simulink model "QueuingSys"  (R2019a)
settings: Solver=VariableStepAuto  StartTime=0.0  StopTime=100  RelTol=1e-3  EnableMultiTasking=on
undefined symbols (not defined in the file or in its folder): m, n
(part 1 of 5)
settings Model: Creator=The MathWorks, Inc.  LastModifiedBy=Mojzar
settings DataIOCC: LimitDataPoints=on  SaveFormat=Array  ReturnWorkspaceOutputs=off
settings OptimizationCC: LifeSpan=inf
settings DebuggingCC: AllowSymbolicDim=off  SFUnexpectedBacktrackingDiag=warning  SFNoUnconditionalDefaultTransitionDiag=warning  SFExecutionAtInitializationDiag=none  ArithmeticOperatorsInVariantConditions=warning
settings ModelReferenceCC: PropagateSignalLabelsOutOfModel=off
settings SFSimCC: SimUseLocalCustomCode=off
settings RTWCC: RTWUseLocalCustomCode=off
settings CodeAppCC: StateflowObjectComments=on
settings GRTTargetCC: TargetLangStandard=C89/C90 (ANSI)  GeneratePreprocessorConditionals=Disable all
settings ConfigComp: CovMetricSettings=dw  CovHtmlReporting=on  CovSaveCumulativeToWorkspaceVar=on  CovSaveSingleToWorkspaceVar=on  CovExternalEMLEnable=off  CovSFcnEnable=off

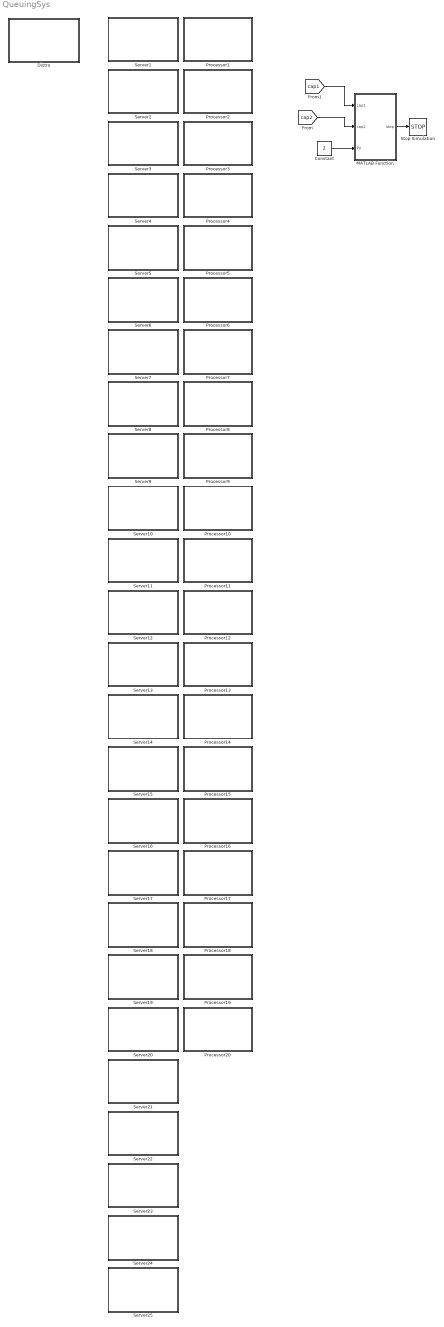
== system QueuingSys ==
  Constant : Constant  Value=2  SampleTime=-1
  Distro : Subsystem
  MATLAB Function : MATLAB Function  TreatAsAtomicUnit=on
  Processor1 : Subsystem
  Processor10 : Subsystem
  Processor11 : Subsystem
  Processor12 : Subsystem
  Processor13 : Subsystem
  Processor14 : Subsystem
  Processor15 : Subsystem
  Processor16 : Subsystem
  Processor17 : Subsystem
  Processor18 : Subsystem
  Processor19 : Subsystem
  Processor2 : Subsystem
  Processor20 : Subsystem
  Processor3 : Subsystem
  Processor4 : Subsystem
  Processor5 : Subsystem
  Processor6 : Subsystem
  Processor7 : Subsystem
  Processor8 : Subsystem
  Processor9 : Subsystem
  Server1 : Subsystem
  Server10 : Subsystem
  Server11 : Subsystem
  Server12 : Subsystem
  Server13 : Subsystem
  Server14 : Subsystem
  Server15 : Subsystem
  Server16 : Subsystem
  Server17 : Subsystem
  Server18 : Subsystem
  Server19 : Subsystem
  Server2 : Subsystem
  Server20 : Subsystem
  Server21 : Subsystem
  Server22 : Subsystem
  Server23 : Subsystem
  Server24 : Subsystem
  Server25 : Subsystem
  Server3 : Subsystem
  Server4 : Subsystem
  Server5 : Subsystem
  Server6 : Subsystem
  Server7 : Subsystem
  Server8 : Subsystem
  Server9 : Subsystem
  Stop Simulation : Stop
  wires:
  [cap2] -> MATLAB Function/2(cap2)
  [cap1] -> MATLAB Function/1(cap1)
  MATLAB Function/1(stop) -> Stop Simulation/1
  Constant/1 -> MATLAB Function/3(Pn)

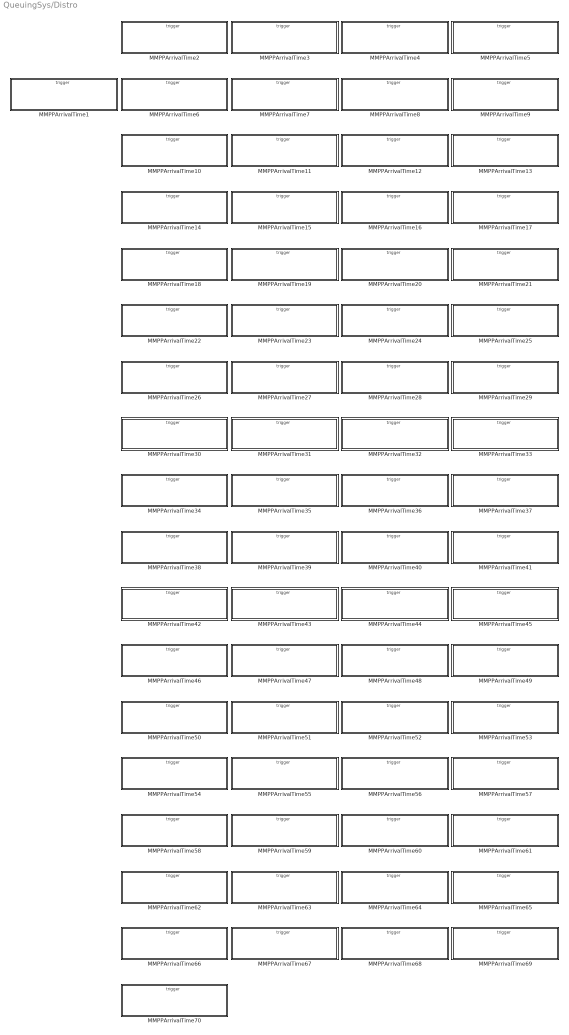
== system QueuingSys/Distro ==
  MMPPArrivalTime1 : Subsystem  TreatAsAtomicUnit=on
  MMPPArrivalTime10 : Subsystem  TreatAsAtomicUnit=on
  MMPPArrivalTime11 : Subsystem  TreatAsAtomicUnit=on
  MMPPArrivalTime12 : Subsystem  TreatAsAtomicUnit=on
  MMPPArrivalTime13 : Subsystem  TreatAsAtomicUnit=on
  MMPPArrivalTime14 : Subsystem  TreatAsAtomicUnit=on
  MMPPArrivalTime15 : Subsystem  TreatAsAtomicUnit=on
  MMPPArrivalTime16 : Subsystem  TreatAsAtomicUnit=on
  MMPPArrivalTime17 : Subsystem  TreatAsAtomicUnit=on
  MMPPArrivalTime18 : Subsystem  TreatAsAtomicUnit=on
  MMPPArrivalTime19 : Subsystem  TreatAsAtomicUnit=on
  MMPPArrivalTime2 : Subsystem  TreatAsAtomicUnit=on
  MMPPArrivalTime20 : Subsystem  TreatAsAtomicUnit=on
  MMPPArrivalTime21 : Subsystem  TreatAsAtomicUnit=on
  MMPPArrivalTime22 : Subsystem  TreatAsAtomicUnit=on
  MMPPArrivalTime23 : Subsystem  TreatAsAtomicUnit=on
  MMPPArrivalTime24 : Subsystem  TreatAsAtomicUnit=on
  MMPPArrivalTime25 : Subsystem  TreatAsAtomicUnit=on
  MMPPArrivalTime26 : Subsystem  TreatAsAtomicUnit=on
  MMPPArrivalTime27 : Subsystem  TreatAsAtomicUnit=on
  MMPPArrivalTime28 : Subsystem  TreatAsAtomicUnit=on
  MMPPArrivalTime29 : Subsystem  TreatAsAtomicUnit=on
  MMPPArrivalTime3 : Subsystem  TreatAsAtomicUnit=on
  MMPPArrivalTime30 : Subsystem  TreatAsAtomicUnit=on
  MMPPArrivalTime31 : Subsystem  TreatAsAtomicUnit=on
  MMPPArrivalTime32 : Subsystem  TreatAsAtomicUnit=on
  MMPPArrivalTime33 : Subsystem  TreatAsAtomicUnit=on
  MMPPArrivalTime34 : Subsystem  TreatAsAtomicUnit=on
  MMPPArrivalTime35 : Subsystem  TreatAsAtomicUnit=on
  MMPPArrivalTime36 : Subsystem  TreatAsAtomicUnit=on
  MMPPArrivalTime37 : Subsystem  TreatAsAtomicUnit=on
  MMPPArrivalTime38 : Subsystem  TreatAsAtomicUnit=on
  MMPPArrivalTime39 : Subsystem  TreatAsAtomicUnit=on
  MMPPArrivalTime4 : Subsystem  TreatAsAtomicUnit=on
  MMPPArrivalTime40 : Subsystem  TreatAsAtomicUnit=on
  MMPPArrivalTime41 : Subsystem  TreatAsAtomicUnit=on
  MMPPArrivalTime42 : Subsystem  TreatAsAtomicUnit=on
  MMPPArrivalTime43 : Subsystem  TreatAsAtomicUnit=on
  MMPPArrivalTime44 : Subsystem  TreatAsAtomicUnit=on
  MMPPArrivalTime45 : Subsystem  TreatAsAtomicUnit=on
  MMPPArrivalTime46 : Subsystem  TreatAsAtomicUnit=on
  MMPPArrivalTime47 : Subsystem  TreatAsAtomicUnit=on
  MMPPArrivalTime48 : Subsystem  TreatAsAtomicUnit=on
  MMPPArrivalTime49 : Subsystem  TreatAsAtomicUnit=on
  MMPPArrivalTime5 : Subsystem  TreatAsAtomicUnit=on
  MMPPArrivalTime50 : Subsystem  TreatAsAtomicUnit=on
  MMPPArrivalTime51 : Subsystem  TreatAsAtomicUnit=on
  MMPPArrivalTime52 : Subsystem  TreatAsAtomicUnit=on
  MMPPArrivalTime53 : Subsystem  TreatAsAtomicUnit=on
  MMPPArrivalTime54 : Subsystem  TreatAsAtomicUnit=on
  MMPPArrivalTime55 : Subsystem  TreatAsAtomicUnit=on
  MMPPArrivalTime56 : Subsystem  TreatAsAtomicUnit=on
  MMPPArrivalTime57 : Subsystem  TreatAsAtomicUnit=on
  MMPPArrivalTime58 : Subsystem  TreatAsAtomicUnit=on
  MMPPArrivalTime59 : Subsystem  TreatAsAtomicUnit=on
  MMPPArrivalTime6 : Subsystem  TreatAsAtomicUnit=on
  MMPPArrivalTime60 : Subsystem  TreatAsAtomicUnit=on
  MMPPArrivalTime61 : Subsystem  TreatAsAtomicUnit=on
  MMPPArrivalTime62 : Subsystem  TreatAsAtomicUnit=on
  MMPPArrivalTime63 : Subsystem  TreatAsAtomicUnit=on
  MMPPArrivalTime64 : Subsystem  TreatAsAtomicUnit=on
  MMPPArrivalTime65 : Subsystem  TreatAsAtomicUnit=on
  MMPPArrivalTime66 : Subsystem  TreatAsAtomicUnit=on
  MMPPArrivalTime67 : Subsystem  TreatAsAtomicUnit=on
  MMPPArrivalTime68 : Subsystem  TreatAsAtomicUnit=on
  MMPPArrivalTime69 : Subsystem  TreatAsAtomicUnit=on
  MMPPArrivalTime7 : Subsystem  TreatAsAtomicUnit=on
  MMPPArrivalTime70 : Subsystem  TreatAsAtomicUnit=on
  MMPPArrivalTime8 : Subsystem  TreatAsAtomicUnit=on
  MMPPArrivalTime9 : Subsystem  TreatAsAtomicUnit=on

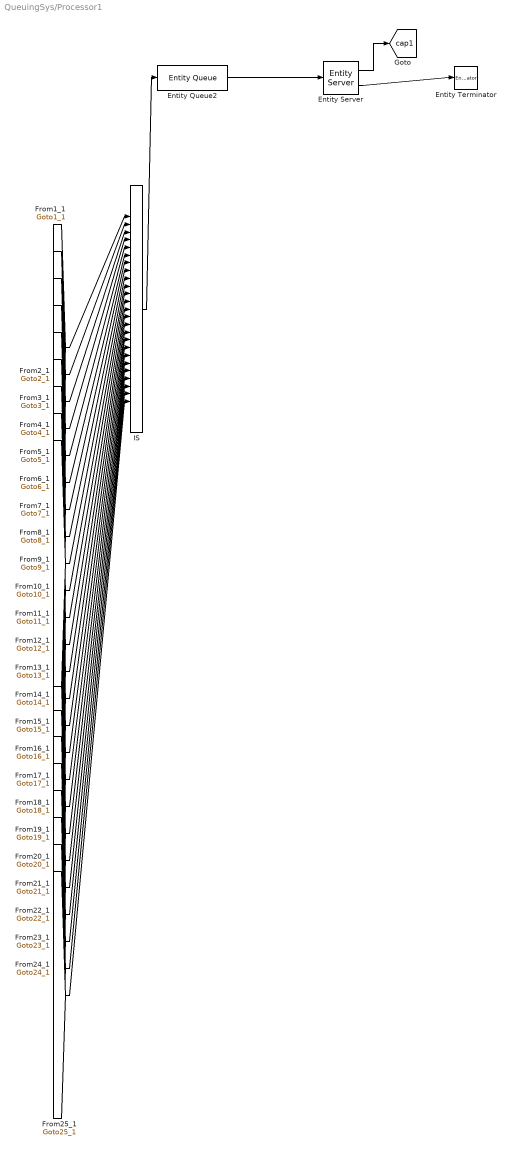
== system QueuingSys/Processor1 ==
  Entity Queue2 : EntityQueue  InputPortMessageModes=m  OutputPortMessageModes=m  Capacity=Inf  MulticastTag=B
      settings: OutputPortMap=o5
  Entity Server : EntityServer  InputPortMessageModes=m  OutputPortMessageModes=n,m  Capacity=4  ServiceTimeSource=MATLAB action  ServiceTimeAction=dt =MMPPArrivalTime51();  NumberEntitiesInBlock=on
      settings: OutputPortMap=o1,o9
  Entity Terminator : EntityTerminator  InputPortMessageModes=m
  IS : EntityInputSwitch  InputPortMessageModes=m,m,m,m,m,m,m,m,m,m,m,m,m,m,m,m,m,m,m,m,m,m,m,m,m  OutputPortMessageModes=m  NumberInputPorts=25
      settings: InputPortMap=u1,u2,u3,u4,u5,u6,u7,u8,u9,u10,u11,u12,u13,u14,u15,u16,u17,u18,u19,u20,u21,u22,u23,u24,u25
  tag scope: cap1=global
  wires:
  IS/1 -> Entity Queue2/1
  Entity Server/2 -> Entity Terminator/1
  Entity Queue2/1 -> Entity Server/1
  [Goto1_1] -> IS/1
  [Goto2_1] -> IS/2
  [Goto3_1] -> IS/3
  [Goto4_1] -> IS/4
  [Goto5_1] -> IS/5
  [Goto6_1] -> IS/6
  [Goto7_1] -> IS/7
  [Goto8_1] -> IS/8
  [Goto9_1] -> IS/9
  [Goto10_1] -> IS/10
  [Goto11_1] -> IS/11
  [Goto12_1] -> IS/12
  [Goto13_1] -> IS/13
  [Goto14_1] -> IS/14
  [Goto15_1] -> IS/15
  [Goto16_1] -> IS/16
  [Goto17_1] -> IS/17
  [Goto18_1] -> IS/18
  [Goto19_1] -> IS/19
  [Goto20_1] -> IS/20
  [Goto21_1] -> IS/21
  [Goto22_1] -> IS/22
  [Goto23_1] -> IS/23
  [Goto24_1] -> IS/24
  [Goto25_1] -> IS/25
  Entity Server/1 -> [cap1]

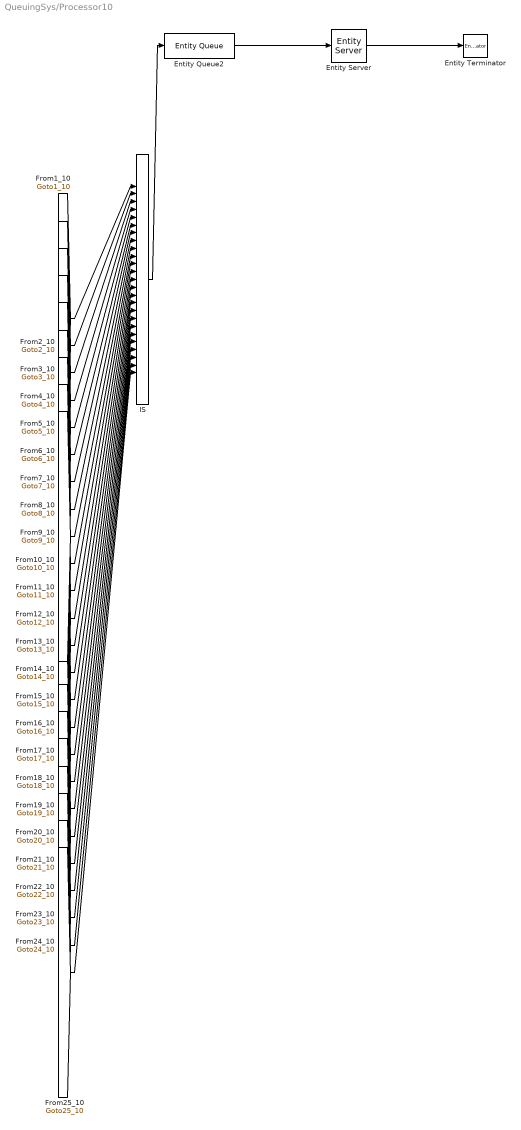
== system QueuingSys/Processor10 ==
  Entity Queue2 : EntityQueue  InputPortMessageModes=m  OutputPortMessageModes=m  Capacity=Inf  MulticastTag=B
      settings: OutputPortMap=o5
  Entity Server : EntityServer  InputPortMessageModes=m  OutputPortMessageModes=m  Capacity=3  ServiceTimeSource=MATLAB action  ServiceTimeAction=dt =MMPPArrivalTime60();
  Entity Terminator : EntityTerminator  InputPortMessageModes=m
  IS : EntityInputSwitch  InputPortMessageModes=m,m,m,m,m,m,m,m,m,m,m,m,m,m,m,m,m,m,m,m,m,m,m,m,m  OutputPortMessageModes=m  NumberInputPorts=25
      settings: InputPortMap=u1,u2,u3,u4,u5,u6,u7,u8,u9,u10,u11,u12,u13,u14,u15,u16,u17,u18,u19,u20,u21,u22,u23,u24,u25
  wires:
  Entity Queue2/1 -> Entity Server/1
  Entity Server/1 -> Entity Terminator/1
  IS/1 -> Entity Queue2/1
  [Goto1_10] -> IS/1
  [Goto2_10] -> IS/2
  [Goto3_10] -> IS/3
  [Goto4_10] -> IS/4
  [Goto5_10] -> IS/5
  [Goto6_10] -> IS/6
  [Goto7_10] -> IS/7
  [Goto8_10] -> IS/8
  [Goto9_10] -> IS/9
  [Goto10_10] -> IS/10
  [Goto11_10] -> IS/11
  [Goto12_10] -> IS/12
  [Goto13_10] -> IS/13
  [Goto14_10] -> IS/14
  [Goto15_10] -> IS/15
  [Goto16_10] -> IS/16
  [Goto17_10] -> IS/17
  [Goto18_10] -> IS/18
  [Goto19_10] -> IS/19
  [Goto20_10] -> IS/20
  [Goto21_10] -> IS/21
  [Goto22_10] -> IS/22
  [Goto23_10] -> IS/23
  [Goto24_10] -> IS/24
  [Goto25_10] -> IS/25

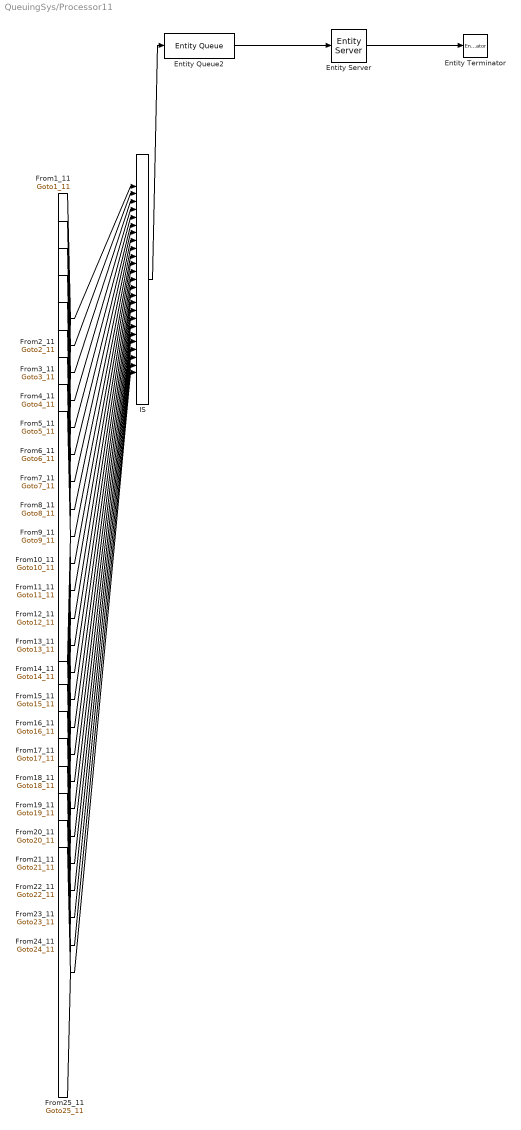
== system QueuingSys/Processor11 ==
  Entity Queue2 : EntityQueue  InputPortMessageModes=m  OutputPortMessageModes=m  Capacity=Inf  MulticastTag=B
      settings: OutputPortMap=o5
  Entity Server : EntityServer  InputPortMessageModes=m  OutputPortMessageModes=m  Capacity=3  ServiceTimeSource=MATLAB action  ServiceTimeAction=dt =MMPPArrivalTime61();
  Entity Terminator : EntityTerminator  InputPortMessageModes=m
  IS : EntityInputSwitch  InputPortMessageModes=m,m,m,m,m,m,m,m,m,m,m,m,m,m,m,m,m,m,m,m,m,m,m,m,m  OutputPortMessageModes=m  NumberInputPorts=25
      settings: InputPortMap=u1,u2,u3,u4,u5,u6,u7,u8,u9,u10,u11,u12,u13,u14,u15,u16,u17,u18,u19,u20,u21,u22,u23,u24,u25
  wires:
  IS/1 -> Entity Queue2/1
  Entity Server/1 -> Entity Terminator/1
  Entity Queue2/1 -> Entity Server/1
  [Goto1_11] -> IS/1
  [Goto2_11] -> IS/2
  [Goto3_11] -> IS/3
  [Goto4_11] -> IS/4
  [Goto5_11] -> IS/5
  [Goto6_11] -> IS/6
  [Goto7_11] -> IS/7
  [Goto8_11] -> IS/8
  [Goto9_11] -> IS/9
  [Goto10_11] -> IS/10
  [Goto11_11] -> IS/11
  [Goto12_11] -> IS/12
  [Goto13_11] -> IS/13
  [Goto14_11] -> IS/14
  [Goto15_11] -> IS/15
  [Goto16_11] -> IS/16
  [Goto17_11] -> IS/17
  [Goto18_11] -> IS/18
  [Goto19_11] -> IS/19
  [Goto20_11] -> IS/20
  [Goto21_11] -> IS/21
  [Goto22_11] -> IS/22
  [Goto23_11] -> IS/23
  [Goto24_11] -> IS/24
  [Goto25_11] -> IS/25

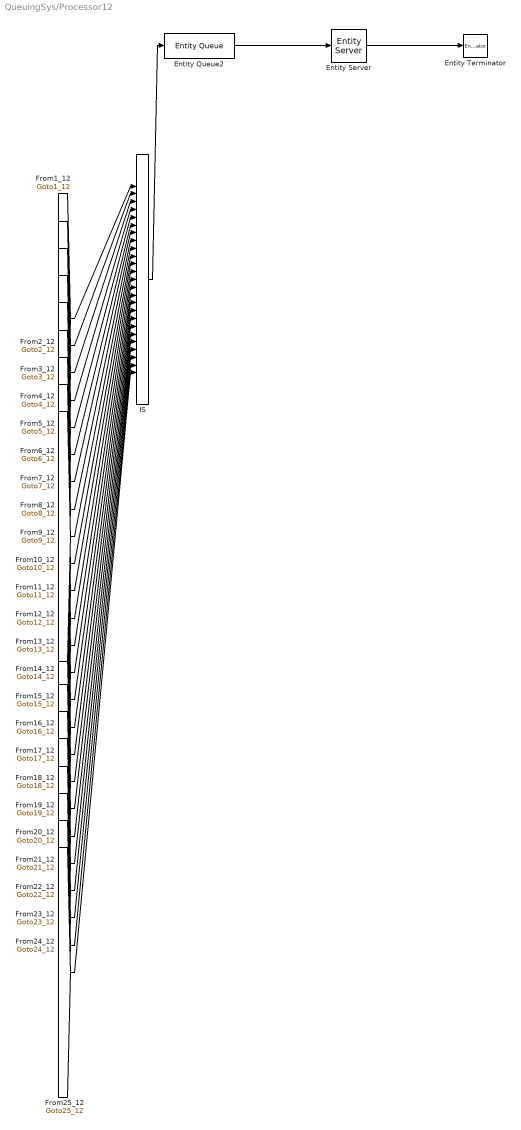
== system QueuingSys/Processor12 ==
  Entity Queue2 : EntityQueue  InputPortMessageModes=m  OutputPortMessageModes=m  Capacity=Inf  MulticastTag=B
      settings: OutputPortMap=o5
  Entity Server : EntityServer  InputPortMessageModes=m  OutputPortMessageModes=m  ServiceTimeSource=MATLAB action  ServiceTimeAction=dt =MMPPArrivalTime62();
  Entity Terminator : EntityTerminator  InputPortMessageModes=m
  IS : EntityInputSwitch  InputPortMessageModes=m,m,m,m,m,m,m,m,m,m,m,m,m,m,m,m,m,m,m,m,m,m,m,m,m  OutputPortMessageModes=m  NumberInputPorts=25
      settings: InputPortMap=u1,u2,u3,u4,u5,u6,u7,u8,u9,u10,u11,u12,u13,u14,u15,u16,u17,u18,u19,u20,u21,u22,u23,u24,u25
  wires:
  Entity Queue2/1 -> Entity Server/1
  Entity Server/1 -> Entity Terminator/1
  IS/1 -> Entity Queue2/1
  [Goto1_12] -> IS/1
  [Goto2_12] -> IS/2
  [Goto3_12] -> IS/3
  [Goto4_12] -> IS/4
  [Goto5_12] -> IS/5
  [Goto6_12] -> IS/6
  [Goto7_12] -> IS/7
  [Goto8_12] -> IS/8
  [Goto9_12] -> IS/9
  [Goto10_12] -> IS/10
  [Goto11_12] -> IS/11
  [Goto12_12] -> IS/12
  [Goto13_12] -> IS/13
  [Goto14_12] -> IS/14
  [Goto15_12] -> IS/15
  [Goto16_12] -> IS/16
  [Goto17_12] -> IS/17
  [Goto18_12] -> IS/18
  [Goto19_12] -> IS/19
  [Goto20_12] -> IS/20
  [Goto21_12] -> IS/21
  [Goto22_12] -> IS/22
  [Goto23_12] -> IS/23
  [Goto24_12] -> IS/24
  [Goto25_12] -> IS/25

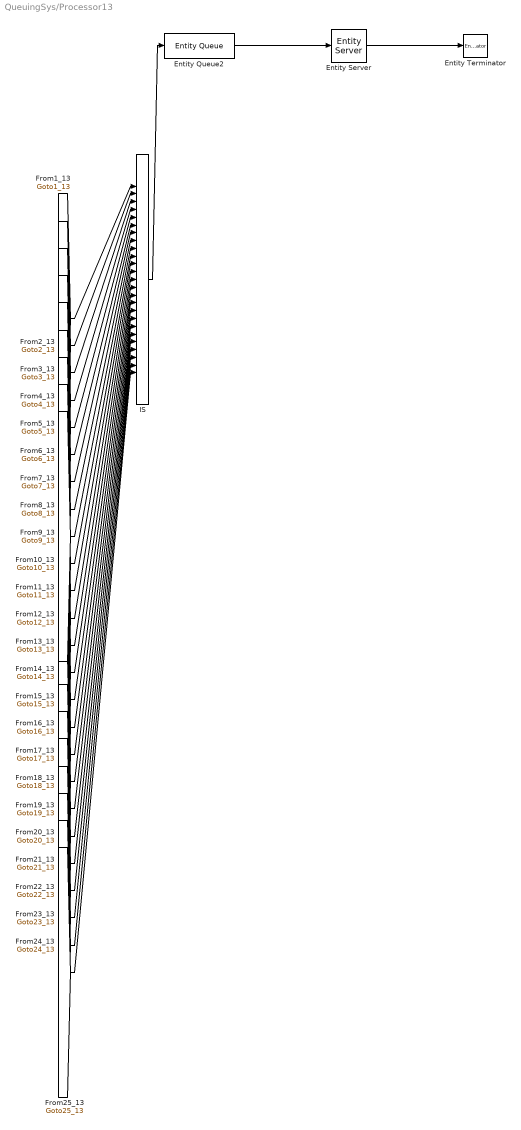
== system QueuingSys/Processor13 ==
  Entity Queue2 : EntityQueue  InputPortMessageModes=m  OutputPortMessageModes=m  Capacity=Inf  MulticastTag=B
      settings: OutputPortMap=o5
  Entity Server : EntityServer  InputPortMessageModes=m  OutputPortMessageModes=m  Capacity=4  ServiceTimeSource=MATLAB action  ServiceTimeAction=dt =MMPPArrivalTime63();
  Entity Terminator : EntityTerminator  InputPortMessageModes=m
  IS : EntityInputSwitch  InputPortMessageModes=m,m,m,m,m,m,m,m,m,m,m,m,m,m,m,m,m,m,m,m,m,m,m,m,m  OutputPortMessageModes=m  NumberInputPorts=25
      settings: InputPortMap=u1,u2,u3,u4,u5,u6,u7,u8,u9,u10,u11,u12,u13,u14,u15,u16,u17,u18,u19,u20,u21,u22,u23,u24,u25
  wires:
  IS/1 -> Entity Queue2/1
  Entity Server/1 -> Entity Terminator/1
  Entity Queue2/1 -> Entity Server/1
  [Goto1_13] -> IS/1
  [Goto2_13] -> IS/2
  [Goto3_13] -> IS/3
  [Goto4_13] -> IS/4
  [Goto5_13] -> IS/5
  [Goto6_13] -> IS/6
  [Goto7_13] -> IS/7
  [Goto8_13] -> IS/8
  [Goto9_13] -> IS/9
  [Goto10_13] -> IS/10
  [Goto11_13] -> IS/11
  [Goto12_13] -> IS/12
  [Goto13_13] -> IS/13
  [Goto14_13] -> IS/14
  [Goto15_13] -> IS/15
  [Goto16_13] -> IS/16
  [Goto17_13] -> IS/17
  [Goto18_13] -> IS/18
  [Goto19_13] -> IS/19
  [Goto20_13] -> IS/20
  [Goto21_13] -> IS/21
  [Goto22_13] -> IS/22
  [Goto23_13] -> IS/23
  [Goto24_13] -> IS/24
  [Goto25_13] -> IS/25

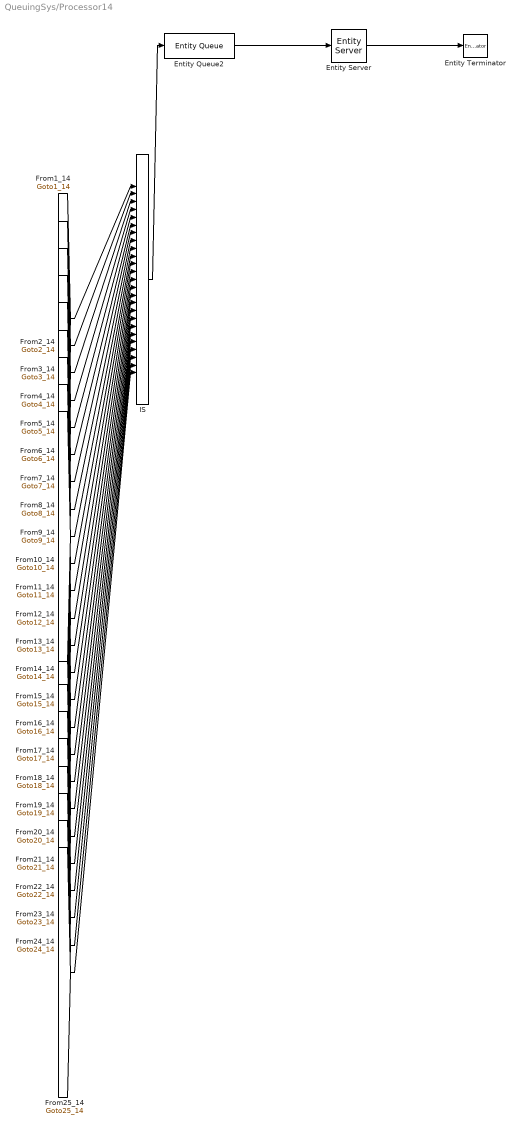
== system QueuingSys/Processor14 ==
  Entity Queue2 : EntityQueue  InputPortMessageModes=m  OutputPortMessageModes=m  Capacity=Inf  MulticastTag=B
      settings: OutputPortMap=o5
  Entity Server : EntityServer  InputPortMessageModes=m  OutputPortMessageModes=m  Capacity=4  ServiceTimeSource=MATLAB action  ServiceTimeAction=dt =MMPPArrivalTime64();
  Entity Terminator : EntityTerminator  InputPortMessageModes=m
  IS : EntityInputSwitch  InputPortMessageModes=m,m,m,m,m,m,m,m,m,m,m,m,m,m,m,m,m,m,m,m,m,m,m,m,m  OutputPortMessageModes=m  NumberInputPorts=25
      settings: InputPortMap=u1,u2,u3,u4,u5,u6,u7,u8,u9,u10,u11,u12,u13,u14,u15,u16,u17,u18,u19,u20,u21,u22,u23,u24,u25
  wires:
  Entity Queue2/1 -> Entity Server/1
  Entity Server/1 -> Entity Terminator/1
  IS/1 -> Entity Queue2/1
  [Goto1_14] -> IS/1
  [Goto2_14] -> IS/2
  [Goto3_14] -> IS/3
  [Goto4_14] -> IS/4
  [Goto5_14] -> IS/5
  [Goto6_14] -> IS/6
  [Goto7_14] -> IS/7
  [Goto8_14] -> IS/8
  [Goto9_14] -> IS/9
  [Goto10_14] -> IS/10
  [Goto11_14] -> IS/11
  [Goto12_14] -> IS/12
  [Goto13_14] -> IS/13
  [Goto14_14] -> IS/14
  [Goto15_14] -> IS/15
  [Goto16_14] -> IS/16
  [Goto17_14] -> IS/17
  [Goto18_14] -> IS/18
  [Goto19_14] -> IS/19
  [Goto20_14] -> IS/20
  [Goto21_14] -> IS/21
  [Goto22_14] -> IS/22
  [Goto23_14] -> IS/23
  [Goto24_14] -> IS/24
  [Goto25_14] -> IS/25

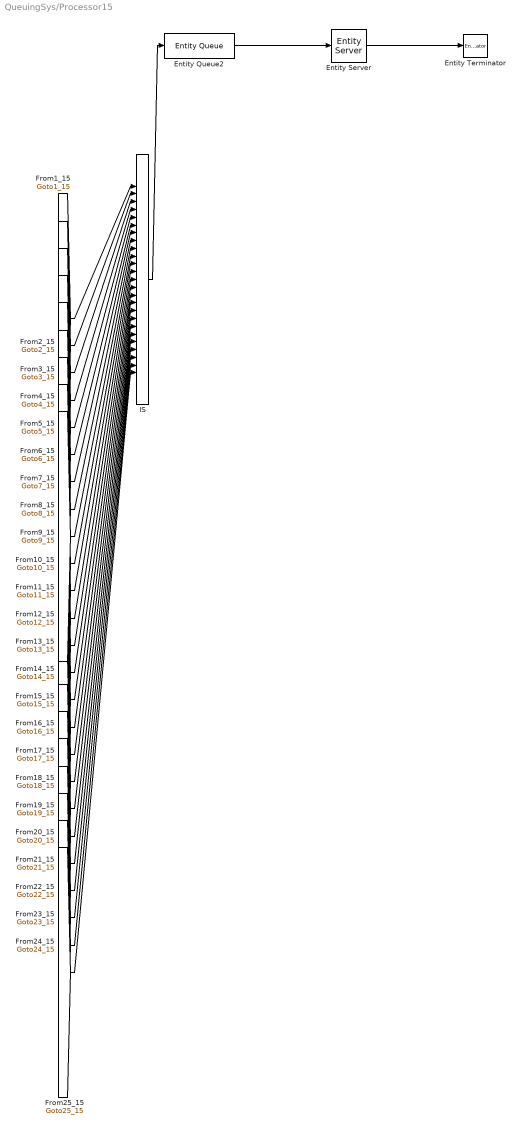
== system QueuingSys/Processor15 ==
  Entity Queue2 : EntityQueue  InputPortMessageModes=m  OutputPortMessageModes=m  Capacity=Inf  MulticastTag=B
      settings: OutputPortMap=o5
  Entity Server : EntityServer  InputPortMessageModes=m  OutputPortMessageModes=m  ServiceTimeSource=MATLAB action  ServiceTimeAction=dt =MMPPArrivalTime65();
  Entity Terminator : EntityTerminator  InputPortMessageModes=m
  IS : EntityInputSwitch  InputPortMessageModes=m,m,m,m,m,m,m,m,m,m,m,m,m,m,m,m,m,m,m,m,m,m,m,m,m  OutputPortMessageModes=m  NumberInputPorts=25
      settings: InputPortMap=u1,u2,u3,u4,u5,u6,u7,u8,u9,u10,u11,u12,u13,u14,u15,u16,u17,u18,u19,u20,u21,u22,u23,u24,u25
  wires:
  IS/1 -> Entity Queue2/1
  Entity Server/1 -> Entity Terminator/1
  Entity Queue2/1 -> Entity Server/1
  [Goto1_15] -> IS/1
  [Goto2_15] -> IS/2
  [Goto3_15] -> IS/3
  [Goto4_15] -> IS/4
  [Goto5_15] -> IS/5
  [Goto6_15] -> IS/6
  [Goto7_15] -> IS/7
  [Goto8_15] -> IS/8
  [Goto9_15] -> IS/9
  [Goto10_15] -> IS/10
  [Goto11_15] -> IS/11
  [Goto12_15] -> IS/12
  [Goto13_15] -> IS/13
  [Goto14_15] -> IS/14
  [Goto15_15] -> IS/15
  [Goto16_15] -> IS/16
  [Goto17_15] -> IS/17
  [Goto18_15] -> IS/18
  [Goto19_15] -> IS/19
  [Goto20_15] -> IS/20
  [Goto21_15] -> IS/21
  [Goto22_15] -> IS/22
  [Goto23_15] -> IS/23
  [Goto24_15] -> IS/24
  [Goto25_15] -> IS/25

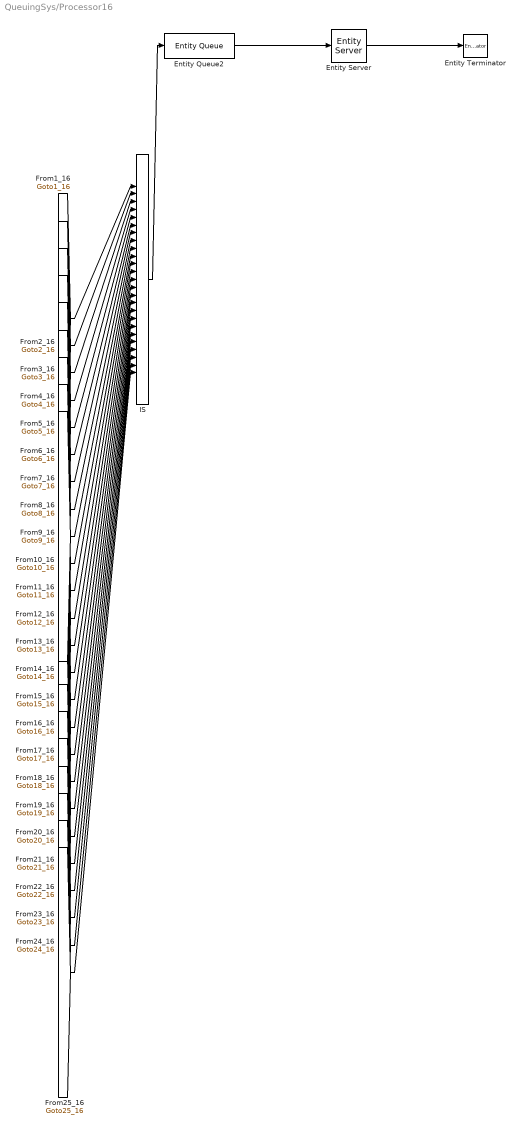
== system QueuingSys/Processor16 ==
  Entity Queue2 : EntityQueue  InputPortMessageModes=m  OutputPortMessageModes=m  Capacity=Inf  MulticastTag=B
      settings: OutputPortMap=o5
  Entity Server : EntityServer  InputPortMessageModes=m  OutputPortMessageModes=m  Capacity=1  ServiceTimeSource=MATLAB action  ServiceTimeAction=dt =MMPPArrivalTime66();
  Entity Terminator : EntityTerminator  InputPortMessageModes=m
  IS : EntityInputSwitch  InputPortMessageModes=m,m,m,m,m,m,m,m,m,m,m,m,m,m,m,m,m,m,m,m,m,m,m,m,m  OutputPortMessageModes=m  NumberInputPorts=25
      settings: InputPortMap=u1,u2,u3,u4,u5,u6,u7,u8,u9,u10,u11,u12,u13,u14,u15,u16,u17,u18,u19,u20,u21,u22,u23,u24,u25
  wires:
  Entity Queue2/1 -> Entity Server/1
  Entity Server/1 -> Entity Terminator/1
  IS/1 -> Entity Queue2/1
  [Goto1_16] -> IS/1
  [Goto2_16] -> IS/2
  [Goto3_16] -> IS/3
  [Goto4_16] -> IS/4
  [Goto5_16] -> IS/5
  [Goto6_16] -> IS/6
  [Goto7_16] -> IS/7
  [Goto8_16] -> IS/8
  [Goto9_16] -> IS/9
  [Goto10_16] -> IS/10
  [Goto11_16] -> IS/11
  [Goto12_16] -> IS/12
  [Goto13_16] -> IS/13
  [Goto14_16] -> IS/14
  [Goto15_16] -> IS/15
  [Goto16_16] -> IS/16
  [Goto17_16] -> IS/17
  [Goto18_16] -> IS/18
  [Goto19_16] -> IS/19
  [Goto20_16] -> IS/20
  [Goto21_16] -> IS/21
  [Goto22_16] -> IS/22
  [Goto23_16] -> IS/23
  [Goto24_16] -> IS/24
  [Goto25_16] -> IS/25

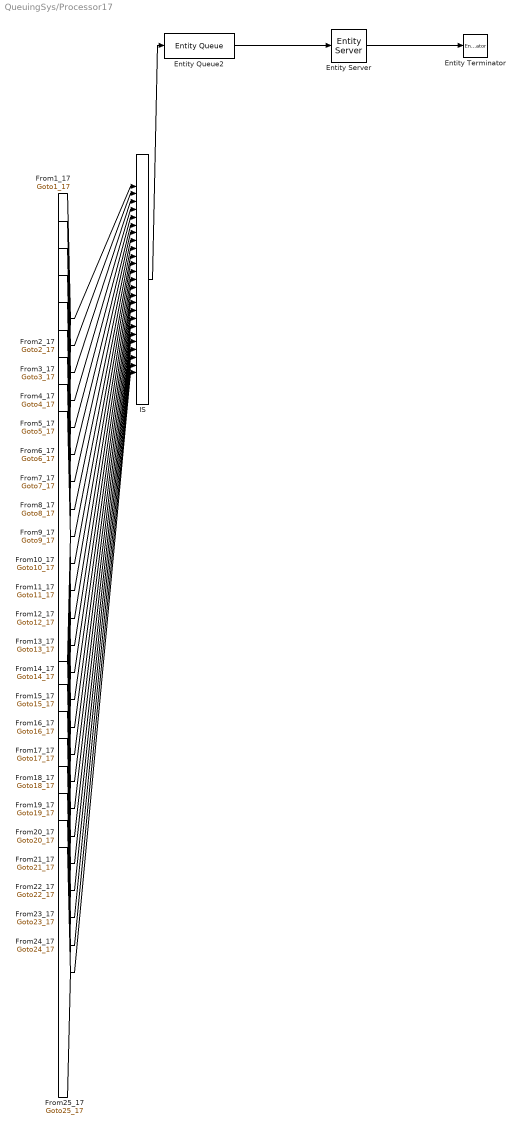
== system QueuingSys/Processor17 ==
  Entity Queue2 : EntityQueue  InputPortMessageModes=m  OutputPortMessageModes=m  Capacity=Inf  MulticastTag=B
      settings: OutputPortMap=o5
  Entity Server : EntityServer  InputPortMessageModes=m  OutputPortMessageModes=m  Capacity=2  ServiceTimeSource=MATLAB action  ServiceTimeAction=dt =MMPPArrivalTime67();
  Entity Terminator : EntityTerminator  InputPortMessageModes=m
  IS : EntityInputSwitch  InputPortMessageModes=m,m,m,m,m,m,m,m,m,m,m,m,m,m,m,m,m,m,m,m,m,m,m,m,m  OutputPortMessageModes=m  NumberInputPorts=25
      settings: InputPortMap=u1,u2,u3,u4,u5,u6,u7,u8,u9,u10,u11,u12,u13,u14,u15,u16,u17,u18,u19,u20,u21,u22,u23,u24,u25
  wires:
  IS/1 -> Entity Queue2/1
  Entity Server/1 -> Entity Terminator/1
  Entity Queue2/1 -> Entity Server/1
  [Goto1_17] -> IS/1
  [Goto2_17] -> IS/2
  [Goto3_17] -> IS/3
  [Goto4_17] -> IS/4
  [Goto5_17] -> IS/5
  [Goto6_17] -> IS/6
  [Goto7_17] -> IS/7
  [Goto8_17] -> IS/8
  [Goto9_17] -> IS/9
  [Goto10_17] -> IS/10
  [Goto11_17] -> IS/11
  [Goto12_17] -> IS/12
  [Goto13_17] -> IS/13
  [Goto14_17] -> IS/14
  [Goto15_17] -> IS/15
  [Goto16_17] -> IS/16
  [Goto17_17] -> IS/17
  [Goto18_17] -> IS/18
  [Goto19_17] -> IS/19
  [Goto20_17] -> IS/20
  [Goto21_17] -> IS/21
  [Goto22_17] -> IS/22
  [Goto23_17] -> IS/23
  [Goto24_17] -> IS/24
  [Goto25_17] -> IS/25

== system QueuingSys/Processor18 ==
  Entity Queue2 : EntityQueue  InputPortMessageModes=m  OutputPortMessageModes=m  Capacity=Inf  MulticastTag=B
      settings: OutputPortMap=o5
  Entity Server : EntityServer  InputPortMessageModes=m  OutputPortMessageModes=m  Capacity=7  ServiceTimeSource=MATLAB action  ServiceTimeAction=dt =MMPPArrivalTime68();
  Entity Terminator : EntityTerminator  InputPortMessageModes=m
  IS : EntityInputSwitch  InputPortMessageModes=m,m,m,m,m,m,m,m,m,m,m,m,m,m,m,m,m,m,m,m,m,m,m,m,m  OutputPortMessageModes=m  NumberInputPorts=25
      settings: InputPortMap=u1,u2,u3,u4,u5,u6,u7,u8,u9,u10,u11,u12,u13,u14,u15,u16,u17,u18,u19,u20,u21,u22,u23,u24,u25
  wires:
  Entity Queue2/1 -> Entity Server/1
  Entity Server/1 -> Entity Terminator/1
  IS/1 -> Entity Queue2/1
  [Goto1_18] -> IS/1
  [Goto2_18] -> IS/2
  [Goto3_18] -> IS/3
  [Goto4_18] -> IS/4
  [Goto5_18] -> IS/5
  [Goto6_18] -> IS/6
  [Goto7_18] -> IS/7
  [Goto8_18] -> IS/8
  [Goto9_18] -> IS/9
  [Goto10_18] -> IS/10
  [Goto11_18] -> IS/11
  [Goto12_18] -> IS/12
  [Goto13_18] -> IS/13
  [Goto14_18] -> IS/14
  [Goto15_18] -> IS/15
  [Goto16_18] -> IS/16
  [Goto17_18] -> IS/17
  [Goto18_18] -> IS/18
  [Goto19_18] -> IS/19
  [Goto20_18] -> IS/20
  [Goto21_18] -> IS/21
  [Goto22_18] -> IS/22
  [Goto23_18] -> IS/23
  [Goto24_18] -> IS/24
  [Goto25_18] -> IS/25

== system QueuingSys/Processor19 ==
  Entity Queue2 : EntityQueue  InputPortMessageModes=m  OutputPortMessageModes=m  Capacity=Inf  MulticastTag=B
      settings: OutputPortMap=o5
  Entity Server : EntityServer  InputPortMessageModes=m  OutputPortMessageModes=m  ServiceTimeSource=MATLAB action  ServiceTimeAction=dt =MMPPArrivalTime69();
  Entity Terminator : EntityTerminator  InputPortMessageModes=m
  IS : EntityInputSwitch  InputPortMessageModes=m,m,m,m,m,m,m,m,m,m,m,m,m,m,m,m,m,m,m,m,m,m,m,m,m  OutputPortMessageModes=m  NumberInputPorts=25
      settings: InputPortMap=u1,u2,u3,u4,u5,u6,u7,u8,u9,u10,u11,u12,u13,u14,u15,u16,u17,u18,u19,u20,u21,u22,u23,u24,u25
  wires:
  IS/1 -> Entity Queue2/1
  Entity Server/1 -> Entity Terminator/1
  Entity Queue2/1 -> Entity Server/1
  [Goto1_19] -> IS/1
  [Goto2_19] -> IS/2
  [Goto3_19] -> IS/3
  [Goto4_19] -> IS/4
  [Goto5_19] -> IS/5
  [Goto6_19] -> IS/6
  [Goto7_19] -> IS/7
  [Goto8_19] -> IS/8
  [Goto9_19] -> IS/9
  [Goto10_19] -> IS/10
  [Goto11_19] -> IS/11
  [Goto12_19] -> IS/12
  [Goto13_19] -> IS/13
  [Goto14_19] -> IS/14
  [Goto15_19] -> IS/15
  [Goto16_19] -> IS/16
  [Goto17_19] -> IS/17
  [Goto18_19] -> IS/18
  [Goto19_19] -> IS/19
  [Goto20_19] -> IS/20
  [Goto21_19] -> IS/21
  [Goto22_19] -> IS/22
  [Goto23_19] -> IS/23
  [Goto24_19] -> IS/24
  [Goto25_19] -> IS/25

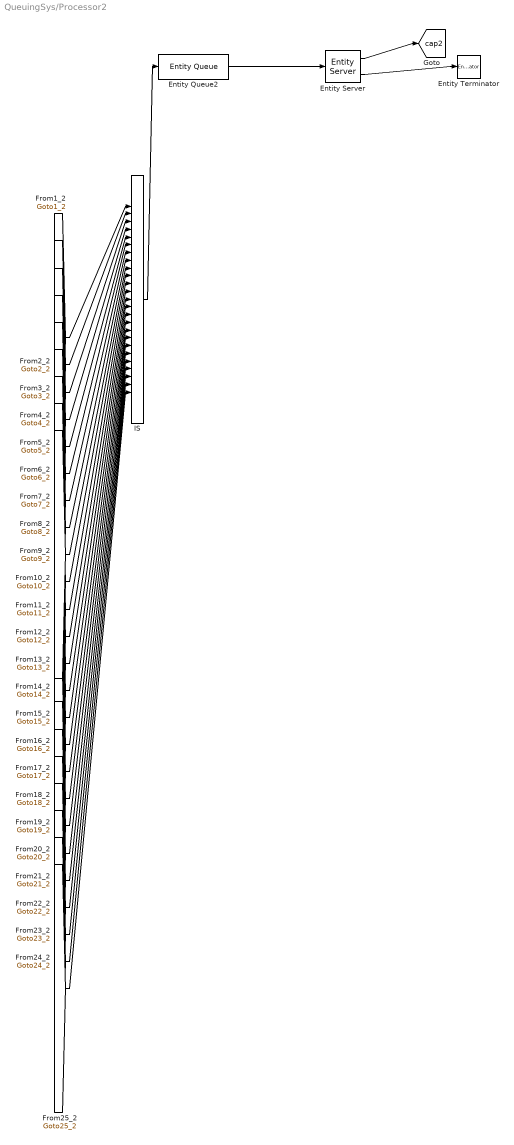
== system QueuingSys/Processor2 ==
  Entity Queue2 : EntityQueue  InputPortMessageModes=m  OutputPortMessageModes=m  Capacity=Inf  MulticastTag=B
      settings: OutputPortMap=o5
  Entity Server : EntityServer  InputPortMessageModes=m  OutputPortMessageModes=n,m  Capacity=3  ServiceTimeSource=MATLAB action  ServiceTimeAction=dt =MMPPArrivalTime52();  NumberEntitiesInBlock=on
      settings: OutputPortMap=o1,o9
  Entity Terminator : EntityTerminator  InputPortMessageModes=m
  IS : EntityInputSwitch  InputPortMessageModes=m,m,m,m,m,m,m,m,m,m,m,m,m,m,m,m,m,m,m,m,m,m,m,m,m  OutputPortMessageModes=m  NumberInputPorts=25
      settings: InputPortMap=u1,u2,u3,u4,u5,u6,u7,u8,u9,u10,u11,u12,u13,u14,u15,u16,u17,u18,u19,u20,u21,u22,u23,u24,u25
  tag scope: cap2=global
  wires:
  Entity Queue2/1 -> Entity Server/1
  Entity Server/2 -> Entity Terminator/1
  IS/1 -> Entity Queue2/1
  [Goto1_2] -> IS/1
  [Goto2_2] -> IS/2
  [Goto3_2] -> IS/3
  [Goto4_2] -> IS/4
  [Goto5_2] -> IS/5
  [Goto6_2] -> IS/6
  [Goto7_2] -> IS/7
  [Goto8_2] -> IS/8
  [Goto9_2] -> IS/9
  [Goto10_2] -> IS/10
  [Goto11_2] -> IS/11
  [Goto12_2] -> IS/12
  [Goto13_2] -> IS/13
  [Goto14_2] -> IS/14
  [Goto15_2] -> IS/15
  [Goto16_2] -> IS/16
  [Goto17_2] -> IS/17
  [Goto18_2] -> IS/18
  [Goto19_2] -> IS/19
  [Goto20_2] -> IS/20
  [Goto21_2] -> IS/21
  [Goto22_2] -> IS/22
  [Goto23_2] -> IS/23
  [Goto24_2] -> IS/24
  [Goto25_2] -> IS/25
  Entity Server/1 -> [cap2]

== system QueuingSys/Processor20 ==
  Entity Queue2 : EntityQueue  InputPortMessageModes=m  OutputPortMessageModes=m  Capacity=Inf  MulticastTag=B
      settings: OutputPortMap=o5
  Entity Server : EntityServer  InputPortMessageModes=m  OutputPortMessageModes=m  Capacity=1  ServiceTimeSource=MATLAB action  ServiceTimeAction=dt =MMPPArrivalTime70();
  Entity Terminator : EntityTerminator  InputPortMessageModes=m
  IS : EntityInputSwitch  InputPortMessageModes=m,m,m,m,m,m,m,m,m,m,m,m,m,m,m,m,m,m,m,m,m,m,m,m,m  OutputPortMessageModes=m  NumberInputPorts=25
      settings: InputPortMap=u1,u2,u3,u4,u5,u6,u7,u8,u9,u10,u11,u12,u13,u14,u15,u16,u17,u18,u19,u20,u21,u22,u23,u24,u25
  wires:
  Entity Queue2/1 -> Entity Server/1
  Entity Server/1 -> Entity Terminator/1
  IS/1 -> Entity Queue2/1
  [Goto1_20] -> IS/1
  [Goto2_20] -> IS/2
  [Goto3_20] -> IS/3
  [Goto4_20] -> IS/4
  [Goto5_20] -> IS/5
  [Goto6_20] -> IS/6
  [Goto7_20] -> IS/7
  [Goto8_20] -> IS/8
  [Goto9_20] -> IS/9
  [Goto10_20] -> IS/10
  [Goto11_20] -> IS/11
  [Goto12_20] -> IS/12
  [Goto13_20] -> IS/13
  [Goto14_20] -> IS/14
  [Goto15_20] -> IS/15
  [Goto16_20] -> IS/16
  [Goto17_20] -> IS/17
  [Goto18_20] -> IS/18
  [Goto19_20] -> IS/19
  [Goto20_20] -> IS/20
  [Goto21_20] -> IS/21
  [Goto22_20] -> IS/22
  [Goto23_20] -> IS/23
  [Goto24_20] -> IS/24
  [Goto25_20] -> IS/25

== system QueuingSys/Processor3 ==
  Entity Queue2 : EntityQueue  InputPortMessageModes=m  OutputPortMessageModes=m  Capacity=Inf  MulticastTag=B
      settings: OutputPortMap=o5
  Entity Server : EntityServer  InputPortMessageModes=m  OutputPortMessageModes=m  Capacity=2  ServiceTimeSource=MATLAB action  ServiceTimeAction=dt =MMPPArrivalTime53();
  Entity Terminator : EntityTerminator  InputPortMessageModes=m
  IS : EntityInputSwitch  InputPortMessageModes=m,m,m,m,m,m,m,m,m,m,m,m,m,m,m,m,m,m,m,m,m,m,m,m,m  OutputPortMessageModes=m  NumberInputPorts=25
      settings: InputPortMap=u1,u2,u3,u4,u5,u6,u7,u8,u9,u10,u11,u12,u13,u14,u15,u16,u17,u18,u19,u20,u21,u22,u23,u24,u25
  wires:
  IS/1 -> Entity Queue2/1
  Entity Server/1 -> Entity Terminator/1
  Entity Queue2/1 -> Entity Server/1
  [Goto1_3] -> IS/1
  [Goto2_3] -> IS/2
  [Goto3_3] -> IS/3
  [Goto4_3] -> IS/4
  [Goto5_3] -> IS/5
  [Goto6_3] -> IS/6
  [Goto7_3] -> IS/7
  [Goto8_3] -> IS/8
  [Goto9_3] -> IS/9
  [Goto10_3] -> IS/10
  [Goto11_3] -> IS/11
  [Goto12_3] -> IS/12
  [Goto13_3] -> IS/13
  [Goto14_3] -> IS/14
  [Goto15_3] -> IS/15
  [Goto16_3] -> IS/16
  [Goto17_3] -> IS/17
  [Goto18_3] -> IS/18
  [Goto19_3] -> IS/19
  [Goto20_3] -> IS/20
  [Goto21_3] -> IS/21
  [Goto22_3] -> IS/22
  [Goto23_3] -> IS/23
  [Goto24_3] -> IS/24
  [Goto25_3] -> IS/25

== system QueuingSys/Processor4 ==
  Entity Queue2 : EntityQueue  InputPortMessageModes=m  OutputPortMessageModes=m  Capacity=Inf  MulticastTag=B
      settings: OutputPortMap=o5
  Entity Server : EntityServer  InputPortMessageModes=m  OutputPortMessageModes=m  Capacity=3  ServiceTimeSource=MATLAB action  ServiceTimeAction=dt =MMPPArrivalTime54();
  Entity Terminator : EntityTerminator  InputPortMessageModes=m
  IS : EntityInputSwitch  InputPortMessageModes=m,m,m,m,m,m,m,m,m,m,m,m,m,m,m,m,m,m,m,m,m,m,m,m,m  OutputPortMessageModes=m  NumberInputPorts=25
      settings: InputPortMap=u1,u2,u3,u4,u5,u6,u7,u8,u9,u10,u11,u12,u13,u14,u15,u16,u17,u18,u19,u20,u21,u22,u23,u24,u25
  wires:
  Entity Queue2/1 -> Entity Server/1
  Entity Server/1 -> Entity Terminator/1
  IS/1 -> Entity Queue2/1
  [Goto1_4] -> IS/1
  [Goto2_4] -> IS/2
  [Goto3_4] -> IS/3
  [Goto4_4] -> IS/4
  [Goto5_4] -> IS/5
  [Goto6_4] -> IS/6
  [Goto7_4] -> IS/7
  [Goto8_4] -> IS/8
  [Goto9_4] -> IS/9
  [Goto10_4] -> IS/10
  [Goto11_4] -> IS/11
  [Goto12_4] -> IS/12
  [Goto13_4] -> IS/13
  [Goto14_4] -> IS/14
  [Goto15_4] -> IS/15
  [Goto16_4] -> IS/16
  [Goto17_4] -> IS/17
  [Goto18_4] -> IS/18
  [Goto19_4] -> IS/19
  [Goto20_4] -> IS/20
  [Goto21_4] -> IS/21
  [Goto22_4] -> IS/22
  [Goto23_4] -> IS/23
  [Goto24_4] -> IS/24
  [Goto25_4] -> IS/25

== system QueuingSys/Processor5 ==
  Entity Queue2 : EntityQueue  InputPortMessageModes=m  OutputPortMessageModes=m  Capacity=Inf  MulticastTag=B
      settings: OutputPortMap=o5
  Entity Server : EntityServer  InputPortMessageModes=m  OutputPortMessageModes=m  Capacity=6  ServiceTimeSource=MATLAB action  ServiceTimeAction=dt =MMPPArrivalTime55();
  Entity Terminator : EntityTerminator  InputPortMessageModes=m
  IS : EntityInputSwitch  InputPortMessageModes=m,m,m,m,m,m,m,m,m,m,m,m,m,m,m,m,m,m,m,m,m,m,m,m,m  OutputPortMessageModes=m  NumberInputPorts=25
      settings: InputPortMap=u1,u2,u3,u4,u5,u6,u7,u8,u9,u10,u11,u12,u13,u14,u15,u16,u17,u18,u19,u20,u21,u22,u23,u24,u25
  wires:
  IS/1 -> Entity Queue2/1
  Entity Server/1 -> Entity Terminator/1
  Entity Queue2/1 -> Entity Server/1
  [Goto1_5] -> IS/1
  [Goto2_5] -> IS/2
  [Goto3_5] -> IS/3
  [Goto4_5] -> IS/4
  [Goto5_5] -> IS/5
  [Goto6_5] -> IS/6
  [Goto7_5] -> IS/7
  [Goto8_5] -> IS/8
  [Goto9_5] -> IS/9
  [Goto10_5] -> IS/10
  [Goto11_5] -> IS/11
  [Goto12_5] -> IS/12
  [Goto13_5] -> IS/13
  [Goto14_5] -> IS/14
  [Goto15_5] -> IS/15
  [Goto16_5] -> IS/16
  [Goto17_5] -> IS/17
  [Goto18_5] -> IS/18
  [Goto19_5] -> IS/19
  [Goto20_5] -> IS/20
  [Goto21_5] -> IS/21
  [Goto22_5] -> IS/22
  [Goto23_5] -> IS/23
  [Goto24_5] -> IS/24
  [Goto25_5] -> IS/25

== system QueuingSys/Processor6 ==
  Entity Queue2 : EntityQueue  InputPortMessageModes=m  OutputPortMessageModes=m  Capacity=Inf  MulticastTag=B
      settings: OutputPortMap=o5
  Entity Server : EntityServer  InputPortMessageModes=m  OutputPortMessageModes=m  Capacity=6  ServiceTimeSource=MATLAB action  ServiceTimeAction=dt =MMPPArrivalTime56();
  Entity Terminator : EntityTerminator  InputPortMessageModes=m
  IS : EntityInputSwitch  InputPortMessageModes=m,m,m,m,m,m,m,m,m,m,m,m,m,m,m,m,m,m,m,m,m,m,m,m,m  OutputPortMessageModes=m  NumberInputPorts=25
      settings: InputPortMap=u1,u2,u3,u4,u5,u6,u7,u8,u9,u10,u11,u12,u13,u14,u15,u16,u17,u18,u19,u20,u21,u22,u23,u24,u25
  wires:
  Entity Queue2/1 -> Entity Server/1
  Entity Server/1 -> Entity Terminator/1
  IS/1 -> Entity Queue2/1
  [Goto1_6] -> IS/1
  [Goto2_6] -> IS/2
  [Goto3_6] -> IS/3
  [Goto4_6] -> IS/4
  [Goto5_6] -> IS/5
  [Goto6_6] -> IS/6
  [Goto7_6] -> IS/7
  [Goto8_6] -> IS/8
  [Goto9_6] -> IS/9
  [Goto10_6] -> IS/10
  [Goto11_6] -> IS/11
  [Goto12_6] -> IS/12
  [Goto13_6] -> IS/13
  [Goto14_6] -> IS/14
  [Goto15_6] -> IS/15
  [Goto16_6] -> IS/16
  [Goto17_6] -> IS/17
  [Goto18_6] -> IS/18
  [Goto19_6] -> IS/19
  [Goto20_6] -> IS/20
  [Goto21_6] -> IS/21
  [Goto22_6] -> IS/22
  [Goto23_6] -> IS/23
  [Goto24_6] -> IS/24
  [Goto25_6] -> IS/25

== system QueuingSys/Processor7 ==
  Entity Queue2 : EntityQueue  InputPortMessageModes=m  OutputPortMessageModes=m  Capacity=Inf  MulticastTag=B
      settings: OutputPortMap=o5
  Entity Server : EntityServer  InputPortMessageModes=m  OutputPortMessageModes=m  Capacity=7  ServiceTimeSource=MATLAB action  ServiceTimeAction=dt =MMPPArrivalTime57();
  Entity Terminator : EntityTerminator  InputPortMessageModes=m
  IS : EntityInputSwitch  InputPortMessageModes=m,m,m,m,m,m,m,m,m,m,m,m,m,m,m,m,m,m,m,m,m,m,m,m,m  OutputPortMessageModes=m  NumberInputPorts=25
      settings: InputPortMap=u1,u2,u3,u4,u5,u6,u7,u8,u9,u10,u11,u12,u13,u14,u15,u16,u17,u18,u19,u20,u21,u22,u23,u24,u25
  wires:
  IS/1 -> Entity Queue2/1
  Entity Server/1 -> Entity Terminator/1
  Entity Queue2/1 -> Entity Server/1
  [Goto1_7] -> IS/1
  [Goto2_7] -> IS/2
  [Goto3_7] -> IS/3
  [Goto4_7] -> IS/4
  [Goto5_7] -> IS/5
  [Goto6_7] -> IS/6
  [Goto7_7] -> IS/7
  [Goto8_7] -> IS/8
  [Goto9_7] -> IS/9
  [Goto10_7] -> IS/10
  [Goto11_7] -> IS/11
  [Goto12_7] -> IS/12
  [Goto13_7] -> IS/13
  [Goto14_7] -> IS/14
  [Goto15_7] -> IS/15
  [Goto16_7] -> IS/16
  [Goto17_7] -> IS/17
  [Goto18_7] -> IS/18
  [Goto19_7] -> IS/19
  [Goto20_7] -> IS/20
  [Goto21_7] -> IS/21
  [Goto22_7] -> IS/22
  [Goto23_7] -> IS/23
  [Goto24_7] -> IS/24
  [Goto25_7] -> IS/25

== system QueuingSys/Processor8 ==
  Entity Queue2 : EntityQueue  InputPortMessageModes=m  OutputPortMessageModes=m  Capacity=Inf  MulticastTag=B
      settings: OutputPortMap=o5
  Entity Server : EntityServer  InputPortMessageModes=m  OutputPortMessageModes=m  Capacity=4  ServiceTimeSource=MATLAB action  ServiceTimeAction=dt =MMPPArrivalTime58();
  Entity Terminator : EntityTerminator  InputPortMessageModes=m
  IS : EntityInputSwitch  InputPortMessageModes=m,m,m,m,m,m,m,m,m,m,m,m,m,m,m,m,m,m,m,m,m,m,m,m,m  OutputPortMessageModes=m  NumberInputPorts=25
      settings: InputPortMap=u1,u2,u3,u4,u5,u6,u7,u8,u9,u10,u11,u12,u13,u14,u15,u16,u17,u18,u19,u20,u21,u22,u23,u24,u25
  wires:
  Entity Queue2/1 -> Entity Server/1
  Entity Server/1 -> Entity Terminator/1
  IS/1 -> Entity Queue2/1
  [Goto1_8] -> IS/1
  [Goto2_8] -> IS/2
  [Goto3_8] -> IS/3
  [Goto4_8] -> IS/4
  [Goto5_8] -> IS/5
  [Goto6_8] -> IS/6
  [Goto7_8] -> IS/7
  [Goto8_8] -> IS/8
  [Goto9_8] -> IS/9
  [Goto10_8] -> IS/10
  [Goto11_8] -> IS/11
  [Goto12_8] -> IS/12
  [Goto13_8] -> IS/13
  [Goto14_8] -> IS/14
  [Goto15_8] -> IS/15
  [Goto16_8] -> IS/16
  [Goto17_8] -> IS/17
  [Goto18_8] -> IS/18
  [Goto19_8] -> IS/19
  [Goto20_8] -> IS/20
  [Goto21_8] -> IS/21
  [Goto22_8] -> IS/22
  [Goto23_8] -> IS/23
  [Goto24_8] -> IS/24
  [Goto25_8] -> IS/25

== system QueuingSys/Processor9 ==
  Entity Queue2 : EntityQueue  InputPortMessageModes=m  OutputPortMessageModes=m  Capacity=Inf  MulticastTag=B
      settings: OutputPortMap=o5
  Entity Server : EntityServer  InputPortMessageModes=m  OutputPortMessageModes=m  ServiceTimeSource=MATLAB action  ServiceTimeAction=dt =MMPPArrivalTime59();
  Entity Terminator : EntityTerminator  InputPortMessageModes=m
  IS : EntityInputSwitch  InputPortMessageModes=m,m,m,m,m,m,m,m,m,m,m,m,m,m,m,m,m,m,m,m,m,m,m,m,m  OutputPortMessageModes=m  NumberInputPorts=25
      settings: InputPortMap=u1,u2,u3,u4,u5,u6,u7,u8,u9,u10,u11,u12,u13,u14,u15,u16,u17,u18,u19,u20,u21,u22,u23,u24,u25
  wires:
  IS/1 -> Entity Queue2/1
  Entity Server/1 -> Entity Terminator/1
  Entity Queue2/1 -> Entity Server/1
  [Goto1_9] -> IS/1
  [Goto2_9] -> IS/2
  [Goto3_9] -> IS/3
  [Goto4_9] -> IS/4
  [Goto5_9] -> IS/5
  [Goto6_9] -> IS/6
  [Goto7_9] -> IS/7
  [Goto8_9] -> IS/8
  [Goto9_9] -> IS/9
  [Goto10_9] -> IS/10
  [Goto11_9] -> IS/11
  [Goto12_9] -> IS/12
  [Goto13_9] -> IS/13
  [Goto14_9] -> IS/14
  [Goto15_9] -> IS/15
  [Goto16_9] -> IS/16
  [Goto17_9] -> IS/17
  [Goto18_9] -> IS/18
  [Goto19_9] -> IS/19
  [Goto20_9] -> IS/20
  [Goto21_9] -> IS/21
  [Goto22_9] -> IS/22
  [Goto23_9] -> IS/23
  [Goto24_9] -> IS/24
  [Goto25_9] -> IS/25

== system QueuingSys/Server1 ==
  Entity Generator1 : EntityGenerator  OutputPortMessageModes=m  TimeSource=MATLAB action  IntergenerationTimeAction=dt =MMPPArrivalTime1();  EntityType=Structured  EntityTypeName=Entity
  Entity Queue1 : EntityQueue  InputPortMessageModes=m  OutputPortMessageModes=m  Capacity=Inf  MulticastTag=B
      settings: OutputPortMap=o5
  Entity Server : EntityServer  InputPortMessageModes=m  OutputPortMessageModes=m  Capacity=2  ServiceTimeSource=MATLAB action  ServiceTimeAction=dt =MMPPArrivalTime2();
  OS : EntityOutputSwitch  InputPortMessageModes=m  OutputPortMessageModes=m,m,m,m,m,m,m,m,m,m,m,m,m,m,m,m,m,m,m,m  NumberOutputPorts=20  SwitchingCriterion=Round robin  SwitchAttributeName=Attribute1
      settings: OutputPortMap=o0,o1,o2,o3,o4,o5,o6,o7,o8,o9,o10,o11,o12,o13,o14,o15,o16,o17,o18,o19
  tag scope: Goto1_10=global, Goto1_11=global, Goto1_12=global, Goto1_13=global, Goto1_14=global, Goto1_15=global, Goto1_16=global, Goto1_17=global, Goto1_18=global, Goto1_19=global, Goto1_1=global, Goto1_20=global, Goto1_2=global, Goto1_3=global, Goto1_4=global, Goto1_5=global, Goto1_6=global, Goto1_7=global, Goto1_8=global, Goto1_9=global
  wires:
  Entity Server/1 -> OS/1
  Entity Generator1/1 -> Entity Queue1/1
  Entity Queue1/1 -> Entity Server/1
  OS/1 -> [Goto1_1]
  OS/2 -> [Goto1_2]
  OS/3 -> [Goto1_3]
  OS/4 -> [Goto1_4]
  OS/5 -> [Goto1_5]
  OS/6 -> [Goto1_6]
  OS/7 -> [Goto1_7]
  OS/8 -> [Goto1_8]
  OS/9 -> [Goto1_9]
  OS/10 -> [Goto1_10]
  OS/11 -> [Goto1_11]
  OS/12 -> [Goto1_12]
  OS/13 -> [Goto1_13]
  OS/14 -> [Goto1_14]
  OS/15 -> [Goto1_15]
  OS/16 -> [Goto1_16]
  OS/17 -> [Goto1_17]
  OS/18 -> [Goto1_18]
  OS/19 -> [Goto1_19]
  OS/20 -> [Goto1_20]

== system QueuingSys/Server10 ==
  Entity Generator1 : EntityGenerator  OutputPortMessageModes=m  TimeSource=MATLAB action  IntergenerationTimeAction=dt =MMPPArrivalTime19();  EntityType=Structured  EntityTypeName=Entity
  Entity Queue1 : EntityQueue  InputPortMessageModes=m  OutputPortMessageModes=m  Capacity=Inf  MulticastTag=B
      settings: OutputPortMap=o5
  Entity Server : EntityServer  InputPortMessageModes=m  OutputPortMessageModes=m  Capacity=2  ServiceTimeSource=MATLAB action  ServiceTimeAction=dt =MMPPArrivalTime20();
  OS : EntityOutputSwitch  InputPortMessageModes=m  OutputPortMessageModes=m,m,m,m,m,m,m,m,m,m,m,m,m,m,m,m,m,m,m,m  NumberOutputPorts=20  SwitchingCriterion=Round robin  SwitchAttributeName=Attribute1
      settings: OutputPortMap=o0,o1,o2,o3,o4,o5,o6,o7,o8,o9,o10,o11,o12,o13,o14,o15,o16,o17,o18,o19
  tag scope: Goto10_10=global, Goto10_11=global, Goto10_12=global, Goto10_13=global, Goto10_14=global, Goto10_15=global, Goto10_16=global, Goto10_17=global, Goto10_18=global, Goto10_19=global, Goto10_1=global, Goto10_20=global, Goto10_2=global, Goto10_3=global, Goto10_4=global, Goto10_5=global, Goto10_6=global, Goto10_7=global, Goto10_8=global, Goto10_9=global
  wires:
  Entity Queue1/1 -> Entity Server/1
  Entity Generator1/1 -> Entity Queue1/1
  Entity Server/1 -> OS/1
  OS/1 -> [Goto10_1]
  OS/2 -> [Goto10_2]
  OS/3 -> [Goto10_3]
  OS/4 -> [Goto10_4]
  OS/5 -> [Goto10_5]
  OS/6 -> [Goto10_6]
  OS/7 -> [Goto10_7]
  OS/8 -> [Goto10_8]
  OS/9 -> [Goto10_9]
  OS/10 -> [Goto10_10]
  OS/11 -> [Goto10_11]
  OS/12 -> [Goto10_12]
  OS/13 -> [Goto10_13]
  OS/14 -> [Goto10_14]
  OS/15 -> [Goto10_15]
  OS/16 -> [Goto10_16]
  OS/17 -> [Goto10_17]
  OS/18 -> [Goto10_18]
  OS/19 -> [Goto10_19]
  OS/20 -> [Goto10_20]

== system QueuingSys/Server11 ==
  Entity Generator1 : EntityGenerator  OutputPortMessageModes=m  TimeSource=MATLAB action  IntergenerationTimeAction=dt =MMPPArrivalTime21();  EntityType=Structured  EntityTypeName=Entity
  Entity Queue1 : EntityQueue  InputPortMessageModes=m  OutputPortMessageModes=m  Capacity=Inf  MulticastTag=B
      settings: OutputPortMap=o5
  Entity Server : EntityServer  InputPortMessageModes=m  OutputPortMessageModes=m  Capacity=6  ServiceTimeSource=MATLAB action  ServiceTimeAction=dt =MMPPArrivalTime22();
  OS : EntityOutputSwitch  InputPortMessageModes=m  OutputPortMessageModes=m,m,m,m,m,m,m,m,m,m,m,m,m,m,m,m,m,m,m,m  NumberOutputPorts=20  SwitchingCriterion=Round robin  SwitchAttributeName=Attribute1
      settings: OutputPortMap=o0,o1,o2,o3,o4,o5,o6,o7,o8,o9,o10,o11,o12,o13,o14,o15,o16,o17,o18,o19
  tag scope: Goto11_10=global, Goto11_11=global, Goto11_12=global, Goto11_13=global, Goto11_14=global, Goto11_15=global, Goto11_16=global, Goto11_17=global, Goto11_18=global, Goto11_19=global, Goto11_1=global, Goto11_20=global, Goto11_2=global, Goto11_3=global, Goto11_4=global, Goto11_5=global, Goto11_6=global, Goto11_7=global, Goto11_8=global, Goto11_9=global
  wires:
  Entity Server/1 -> OS/1
  Entity Generator1/1 -> Entity Queue1/1
  Entity Queue1/1 -> Entity Server/1
  OS/1 -> [Goto11_1]
  OS/2 -> [Goto11_2]
  OS/3 -> [Goto11_3]
  OS/4 -> [Goto11_4]
  OS/5 -> [Goto11_5]
  OS/6 -> [Goto11_6]
  OS/7 -> [Goto11_7]
  OS/8 -> [Goto11_8]
  OS/9 -> [Goto11_9]
  OS/10 -> [Goto11_10]
  OS/11 -> [Goto11_11]
  OS/12 -> [Goto11_12]
  OS/13 -> [Goto11_13]
  OS/14 -> [Goto11_14]
  OS/15 -> [Goto11_15]
  OS/16 -> [Goto11_16]
  OS/17 -> [Goto11_17]
  OS/18 -> [Goto11_18]
  OS/19 -> [Goto11_19]
  OS/20 -> [Goto11_20]

== system QueuingSys/Server12 ==
  Entity Generator1 : EntityGenerator  OutputPortMessageModes=m  TimeSource=MATLAB action  IntergenerationTimeAction=dt =MMPPArrivalTime23();  EntityType=Structured  EntityTypeName=Entity
  Entity Queue1 : EntityQueue  InputPortMessageModes=m  OutputPortMessageModes=m  Capacity=Inf  MulticastTag=B
      settings: OutputPortMap=o5
  Entity Server : EntityServer  InputPortMessageModes=m  OutputPortMessageModes=m  Capacity=2  ServiceTimeSource=MATLAB action  ServiceTimeAction=dt =MMPPArrivalTime24();
  OS : EntityOutputSwitch  InputPortMessageModes=m  OutputPortMessageModes=m,m,m,m,m,m,m,m,m,m,m,m,m,m,m,m,m,m,m,m  NumberOutputPorts=20  SwitchingCriterion=Round robin  SwitchAttributeName=Attribute1
      settings: OutputPortMap=o0,o1,o2,o3,o4,o5,o6,o7,o8,o9,o10,o11,o12,o13,o14,o15,o16,o17,o18,o19
  tag scope: Goto12_10=global, Goto12_11=global, Goto12_12=global, Goto12_13=global, Goto12_14=global, Goto12_15=global, Goto12_16=global, Goto12_17=global, Goto12_18=global, Goto12_19=global, Goto12_1=global, Goto12_20=global, Goto12_2=global, Goto12_3=global, Goto12_4=global, Goto12_5=global, Goto12_6=global, Goto12_7=global, Goto12_8=global, Goto12_9=global
  wires:
  Entity Queue1/1 -> Entity Server/1
  Entity Generator1/1 -> Entity Queue1/1
  Entity Server/1 -> OS/1
  OS/1 -> [Goto12_1]
  OS/2 -> [Goto12_2]
  OS/3 -> [Goto12_3]
  OS/4 -> [Goto12_4]
  OS/5 -> [Goto12_5]
  OS/6 -> [Goto12_6]
  OS/7 -> [Goto12_7]
  OS/8 -> [Goto12_8]
  OS/9 -> [Goto12_9]
  OS/10 -> [Goto12_10]
  OS/11 -> [Goto12_11]
  OS/12 -> [Goto12_12]
  OS/13 -> [Goto12_13]
  OS/14 -> [Goto12_14]
  OS/15 -> [Goto12_15]
  OS/16 -> [Goto12_16]
  OS/17 -> [Goto12_17]
  OS/18 -> [Goto12_18]
  OS/19 -> [Goto12_19]
  OS/20 -> [Goto12_20]

== system QueuingSys/Server13 ==
  Entity Generator1 : EntityGenerator  OutputPortMessageModes=m  TimeSource=MATLAB action  IntergenerationTimeAction=dt =MMPPArrivalTime25();  EntityType=Structured  EntityTypeName=Entity
  Entity Queue1 : EntityQueue  InputPortMessageModes=m  OutputPortMessageModes=m  Capacity=Inf  MulticastTag=B
      settings: OutputPortMap=o5
  Entity Server : EntityServer  InputPortMessageModes=m  OutputPortMessageModes=m  ServiceTimeSource=MATLAB action  ServiceTimeAction=dt =MMPPArrivalTime26();
  OS : EntityOutputSwitch  InputPortMessageModes=m  OutputPortMessageModes=m,m,m,m,m,m,m,m,m,m,m,m,m,m,m,m,m,m,m,m  NumberOutputPorts=20  SwitchingCriterion=Round robin  SwitchAttributeName=Attribute1
      settings: OutputPortMap=o0,o1,o2,o3,o4,o5,o6,o7,o8,o9,o10,o11,o12,o13,o14,o15,o16,o17,o18,o19
  tag scope: Goto13_10=global, Goto13_11=global, Goto13_12=global, Goto13_13=global, Goto13_14=global, Goto13_15=global, Goto13_16=global, Goto13_17=global, Goto13_18=global, Goto13_19=global, Goto13_1=global, Goto13_20=global, Goto13_2=global, Goto13_3=global, Goto13_4=global, Goto13_5=global, Goto13_6=global, Goto13_7=global, Goto13_8=global, Goto13_9=global
  wires:
  Entity Server/1 -> OS/1
  Entity Generator1/1 -> Entity Queue1/1
  Entity Queue1/1 -> Entity Server/1
  OS/1 -> [Goto13_1]
  OS/2 -> [Goto13_2]
  OS/3 -> [Goto13_3]
  OS/4 -> [Goto13_4]
  OS/5 -> [Goto13_5]
  OS/6 -> [Goto13_6]
  OS/7 -> [Goto13_7]
  OS/8 -> [Goto13_8]
  OS/9 -> [Goto13_9]
  OS/10 -> [Goto13_10]
  OS/11 -> [Goto13_11]
  OS/12 -> [Goto13_12]
  OS/13 -> [Goto13_13]
  OS/14 -> [Goto13_14]
  OS/15 -> [Goto13_15]
  OS/16 -> [Goto13_16]
  OS/17 -> [Goto13_17]
  OS/18 -> [Goto13_18]
  OS/19 -> [Goto13_19]
  OS/20 -> [Goto13_20]

== system QueuingSys/Server14 ==
  Entity Generator1 : EntityGenerator  OutputPortMessageModes=m  TimeSource=MATLAB action  IntergenerationTimeAction=dt =MMPPArrivalTime27();  EntityType=Structured  EntityTypeName=Entity
  Entity Queue1 : EntityQueue  InputPortMessageModes=m  OutputPortMessageModes=m  Capacity=Inf  MulticastTag=B
      settings: OutputPortMap=o5
  Entity Server : EntityServer  InputPortMessageModes=m  OutputPortMessageModes=m  Capacity=3  ServiceTimeSource=MATLAB action  ServiceTimeAction=dt =MMPPArrivalTime28();
  OS : EntityOutputSwitch  InputPortMessageModes=m  OutputPortMessageModes=m,m,m,m,m,m,m,m,m,m,m,m,m,m,m,m,m,m,m,m  NumberOutputPorts=20  SwitchingCriterion=Round robin  SwitchAttributeName=Attribute1
      settings: OutputPortMap=o0,o1,o2,o3,o4,o5,o6,o7,o8,o9,o10,o11,o12,o13,o14,o15,o16,o17,o18,o19
  tag scope: Goto14_10=global, Goto14_11=global, Goto14_12=global, Goto14_13=global, Goto14_14=global, Goto14_15=global, Goto14_16=global, Goto14_17=global, Goto14_18=global, Goto14_19=global, Goto14_1=global, Goto14_20=global, Goto14_2=global, Goto14_3=global, Goto14_4=global, Goto14_5=global, Goto14_6=global, Goto14_7=global, Goto14_8=global, Goto14_9=global
  wires:
  Entity Queue1/1 -> Entity Server/1
  Entity Generator1/1 -> Entity Queue1/1
  Entity Server/1 -> OS/1
  OS/1 -> [Goto14_1]
  OS/2 -> [Goto14_2]
  OS/3 -> [Goto14_3]
  OS/4 -> [Goto14_4]
  OS/5 -> [Goto14_5]
  OS/6 -> [Goto14_6]
  OS/7 -> [Goto14_7]
  OS/8 -> [Goto14_8]
  OS/9 -> [Goto14_9]
  OS/10 -> [Goto14_10]
  OS/11 -> [Goto14_11]
  OS/12 -> [Goto14_12]
  OS/13 -> [Goto14_13]
  OS/14 -> [Goto14_14]
  OS/15 -> [Goto14_15]
  OS/16 -> [Goto14_16]
  OS/17 -> [Goto14_17]
  OS/18 -> [Goto14_18]
  OS/19 -> [Goto14_19]
  OS/20 -> [Goto14_20]

== system QueuingSys/Server15 ==
  Entity Generator1 : EntityGenerator  OutputPortMessageModes=m  TimeSource=MATLAB action  IntergenerationTimeAction=dt =MMPPArrivalTime29();  EntityType=Structured  EntityTypeName=Entity
  Entity Queue1 : EntityQueue  InputPortMessageModes=m  OutputPortMessageModes=m  Capacity=Inf  MulticastTag=B
      settings: OutputPortMap=o5
  Entity Server : EntityServer  InputPortMessageModes=m  OutputPortMessageModes=m  Capacity=6  ServiceTimeSource=MATLAB action  ServiceTimeAction=dt =MMPPArrivalTime30();
  OS : EntityOutputSwitch  InputPortMessageModes=m  OutputPortMessageModes=m,m,m,m,m,m,m,m,m,m,m,m,m,m,m,m,m,m,m,m  NumberOutputPorts=20  SwitchingCriterion=Round robin  SwitchAttributeName=Attribute1
      settings: OutputPortMap=o0,o1,o2,o3,o4,o5,o6,o7,o8,o9,o10,o11,o12,o13,o14,o15,o16,o17,o18,o19
  tag scope: Goto15_10=global, Goto15_11=global, Goto15_12=global, Goto15_13=global, Goto15_14=global, Goto15_15=global, Goto15_16=global, Goto15_17=global, Goto15_18=global, Goto15_19=global, Goto15_1=global, Goto15_20=global, Goto15_2=global, Goto15_3=global, Goto15_4=global, Goto15_5=global, Goto15_6=global, Goto15_7=global, Goto15_8=global, Goto15_9=global
  wires:
  Entity Server/1 -> OS/1
  Entity Generator1/1 -> Entity Queue1/1
  Entity Queue1/1 -> Entity Server/1
  OS/1 -> [Goto15_1]
  OS/2 -> [Goto15_2]
  OS/3 -> [Goto15_3]
  OS/4 -> [Goto15_4]
  OS/5 -> [Goto15_5]
  OS/6 -> [Goto15_6]
  OS/7 -> [Goto15_7]
  OS/8 -> [Goto15_8]
  OS/9 -> [Goto15_9]
  OS/10 -> [Goto15_10]
  OS/11 -> [Goto15_11]
  OS/12 -> [Goto15_12]
  OS/13 -> [Goto15_13]
  OS/14 -> [Goto15_14]
  OS/15 -> [Goto15_15]
  OS/16 -> [Goto15_16]
  OS/17 -> [Goto15_17]
  OS/18 -> [Goto15_18]
  OS/19 -> [Goto15_19]
  OS/20 -> [Goto15_20]

== system QueuingSys/Server16 ==
  Entity Generator1 : EntityGenerator  OutputPortMessageModes=m  TimeSource=MATLAB action  IntergenerationTimeAction=dt =MMPPArrivalTime31();  EntityType=Structured  EntityTypeName=Entity
  Entity Queue1 : EntityQueue  InputPortMessageModes=m  OutputPortMessageModes=m  Capacity=Inf  MulticastTag=B
      settings: OutputPortMap=o5
  Entity Server : EntityServer  InputPortMessageModes=m  OutputPortMessageModes=m  Capacity=1  ServiceTimeSource=MATLAB action  ServiceTimeAction=dt =MMPPArrivalTime32();
  OS : EntityOutputSwitch  InputPortMessageModes=m  OutputPortMessageModes=m,m,m,m,m,m,m,m,m,m,m,m,m,m,m,m,m,m,m,m  NumberOutputPorts=20  SwitchingCriterion=Round robin  SwitchAttributeName=Attribute1
      settings: OutputPortMap=o0,o1,o2,o3,o4,o5,o6,o7,o8,o9,o10,o11,o12,o13,o14,o15,o16,o17,o18,o19
  tag scope: Goto16_10=global, Goto16_11=global, Goto16_12=global, Goto16_13=global, Goto16_14=global, Goto16_15=global, Goto16_16=global, Goto16_17=global, Goto16_18=global, Goto16_19=global, Goto16_1=global, Goto16_20=global, Goto16_2=global, Goto16_3=global, Goto16_4=global, Goto16_5=global, Goto16_6=global, Goto16_7=global, Goto16_8=global, Goto16_9=global
  wires:
  Entity Queue1/1 -> Entity Server/1
  Entity Generator1/1 -> Entity Queue1/1
  Entity Server/1 -> OS/1
  OS/1 -> [Goto16_1]
  OS/2 -> [Goto16_2]
  OS/3 -> [Goto16_3]
  OS/4 -> [Goto16_4]
  OS/5 -> [Goto16_5]
  OS/6 -> [Goto16_6]
  OS/7 -> [Goto16_7]
  OS/8 -> [Goto16_8]
  OS/9 -> [Goto16_9]
  OS/10 -> [Goto16_10]
  OS/11 -> [Goto16_11]
  OS/12 -> [Goto16_12]
  OS/13 -> [Goto16_13]
  OS/14 -> [Goto16_14]
  OS/15 -> [Goto16_15]
  OS/16 -> [Goto16_16]
  OS/17 -> [Goto16_17]
  OS/18 -> [Goto16_18]
  OS/19 -> [Goto16_19]
  OS/20 -> [Goto16_20]

== system QueuingSys/Server17 ==
  Entity Generator1 : EntityGenerator  OutputPortMessageModes=m  TimeSource=MATLAB action  IntergenerationTimeAction=dt =MMPPArrivalTime33();  EntityType=Structured  EntityTypeName=Entity
  Entity Queue1 : EntityQueue  InputPortMessageModes=m  OutputPortMessageModes=m  Capacity=Inf  MulticastTag=B
      settings: OutputPortMap=o5
  Entity Server : EntityServer  InputPortMessageModes=m  OutputPortMessageModes=m  Capacity=2  ServiceTimeSource=MATLAB action  ServiceTimeAction=dt =MMPPArrivalTime34();
  OS : EntityOutputSwitch  InputPortMessageModes=m  OutputPortMessageModes=m,m,m,m,m,m,m,m,m,m,m,m,m,m,m,m,m,m,m,m  NumberOutputPorts=20  SwitchingCriterion=Round robin  SwitchAttributeName=Attribute1
      settings: OutputPortMap=o0,o1,o2,o3,o4,o5,o6,o7,o8,o9,o10,o11,o12,o13,o14,o15,o16,o17,o18,o19
  tag scope: Goto17_10=global, Goto17_11=global, Goto17_12=global, Goto17_13=global, Goto17_14=global, Goto17_15=global, Goto17_16=global, Goto17_17=global, Goto17_18=global, Goto17_19=global, Goto17_1=global, Goto17_20=global, Goto17_2=global, Goto17_3=global, Goto17_4=global, Goto17_5=global, Goto17_6=global, Goto17_7=global, Goto17_8=global, Goto17_9=global
  wires:
  Entity Server/1 -> OS/1
  Entity Generator1/1 -> Entity Queue1/1
  Entity Queue1/1 -> Entity Server/1
  OS/1 -> [Goto17_1]
  OS/2 -> [Goto17_2]
  OS/3 -> [Goto17_3]
  OS/4 -> [Goto17_4]
  OS/5 -> [Goto17_5]
  OS/6 -> [Goto17_6]
  OS/7 -> [Goto17_7]
  OS/8 -> [Goto17_8]
  OS/9 -> [Goto17_9]
  OS/10 -> [Goto17_10]
  OS/11 -> [Goto17_11]
  OS/12 -> [Goto17_12]
  OS/13 -> [Goto17_13]
  OS/14 -> [Goto17_14]
  OS/15 -> [Goto17_15]
  OS/16 -> [Goto17_16]
  OS/17 -> [Goto17_17]
  OS/18 -> [Goto17_18]
  OS/19 -> [Goto17_19]
  OS/20 -> [Goto17_20]
